simulink model "Copy_of_mavsim_chap10_model"  (R2020b)
settings: Solver=ode45  StartTime=0.0  StopTime=400  RelTol=1e-3  EnableMultiTasking=on
InitFcn:
  | param_chap10
undefined symbols (not defined in the file or in its folder): drawPathError, P, path_follow, path_manager_chap10
settings Model: Creator=beard  LastModifiedBy=彭美祥
settings DataIOCC: LimitDataPoints=on  SaveFormat=Array  SignalLoggingSaveFormat=ModelDataLogs  ReturnWorkspaceOutputs=off
settings OptimizationCC: ExpressionDepthLimit=2147483647  InitFltsAndDblsToZero=on  LifeSpan=inf
settings DebuggingCC: UnderspecifiedInitializationDetection=Classic  MergeDetectMultiDrivingBlocksExec=none  SolverPrmCheckMsg=warning  FcnCallInpInsideContextMsg=warning  StateNameClashWarn=warning  SFUnexpectedBacktrackingDiag=warning  SFNoUnconditionalDefaultTransitionDiag=warning  SFExecutionAtInitializationDiag=none  ArithmeticOperatorsInVariantConditions=warning
settings HardwareCC: ProdBitPerPointer=32  ProdBitPerSizeT=32  ProdBitPerPtrDiffT=32  ProdLargestAtomicFloat=None  ProdIntDivRoundTo=Undefined  ProdEndianess=Unspecified  ProdWordSize=32  ProdHWDeviceType=32-bit Generic
settings ModelReferenceCC: PropagateSignalLabelsOutOfModel=off
settings SFSimCC: SimUseLocalCustomCode=off  SimParseCustomCode=off  CustomCodeUndefinedFunction=UseInterfaceOnly
settings RTWCC: RTWUseLocalCustomCode=off
settings CodeAppCC: StateflowObjectComments=on
settings GRTTargetCC: TargetLangStandard=C89/C90 (ANSI)  CombineOutputUpdateFcns=off  GRTInterface=on
settings ConfigComp: CovMetricSettings=dw  CovSaveCumulativeToWorkspaceVar=on  CovSaveSingleToWorkspaceVar=on  CovExternalEMLEnable=off  CovSFcnEnable=off

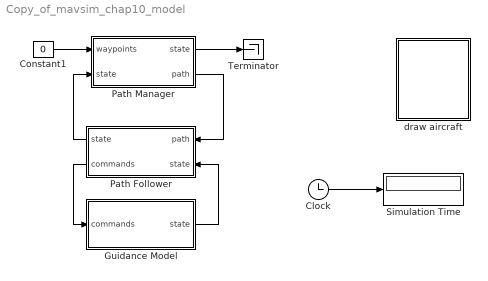
== system Copy_of_mavsim_chap10_model ==
  Clock : Clock
  Constant1 : Constant  Value=0
  Guidance Model : Subsystem
  Path Follower : Subsystem
  Path Manager : Subsystem
  Simulation Time : Display
  Terminator : Terminator
  draw aircraft : Subsystem
      mask Display: image(imread('tv.jpg'))
  wires:
  Clock/1 -> Simulation Time/1
  Path Manager/2(path) -> Path Follower/1(path)
  Path Follower/2(commands) -> Guidance Model/1(commands)
  Guidance Model/1(state) -> Path Follower/2(state)
  Constant1/1 -> Path Manager/1(waypoints)
  Path Follower/1("state ") -> Path Manager/2(state)
  Path Manager/1("state ") -> Terminator/1

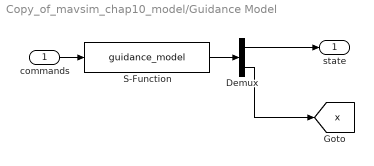
== system Copy_of_mavsim_chap10_model/Guidance Model ==
  commands : Inport
  Demux : Demux  Outputs=[16;12]
  S-Function : S-Function  FunctionName=guidance_model  Parameters=P  SFunctionDeploymentMode=off  EnableBusSupport=off
  state : Outport
  tag scope: x=global
  wires:
  commands/1 -> S-Function/1
  S-Function/1 -> Demux/1
  Demux/1 -> state/1
  Demux/2 -> [x]

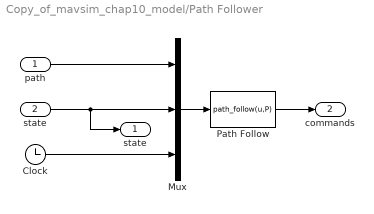
== system Copy_of_mavsim_chap10_model/Path Follower ==
  path : Inport
  state : Inport  Port=2
  Clock : Clock
  Mux : Mux  Inputs=3
  Path Follow : MATLABFcn  MATLABFcn=path_follow(u,P)  OutputDimensions=3  SampleTime=P.Ts
  "state " : Outport
  commands : Outport  Port=2
  wires:
  Path Follow/1 -> commands/1
  Mux/1 -> Path Follow/1
  path/1 -> Mux/1
  Clock/1 -> Mux/3
  state/1 -> Mux/2, "state "/1

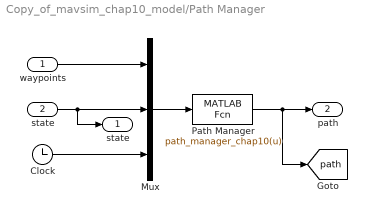
== system Copy_of_mavsim_chap10_model/Path Manager ==
  waypoints : Inport
  state : Inport  Port=2
  Clock : Clock
  Mux : Mux  Inputs=3
  Path Manager : MATLABFcn  MATLABFcn=path_manager_chap10(u)  OutputDimensions=13  SampleTime=P.Ts
  "state " : Outport
  path : Outport  Port=2
  tag scope: path=global
  wires:
  Path Manager/1 -> path/1, [path]
  Mux/1 -> Path Manager/1
  Clock/1 -> Mux/3
  state/1 -> Mux/2, "state "/1
  waypoints/1 -> Mux/1

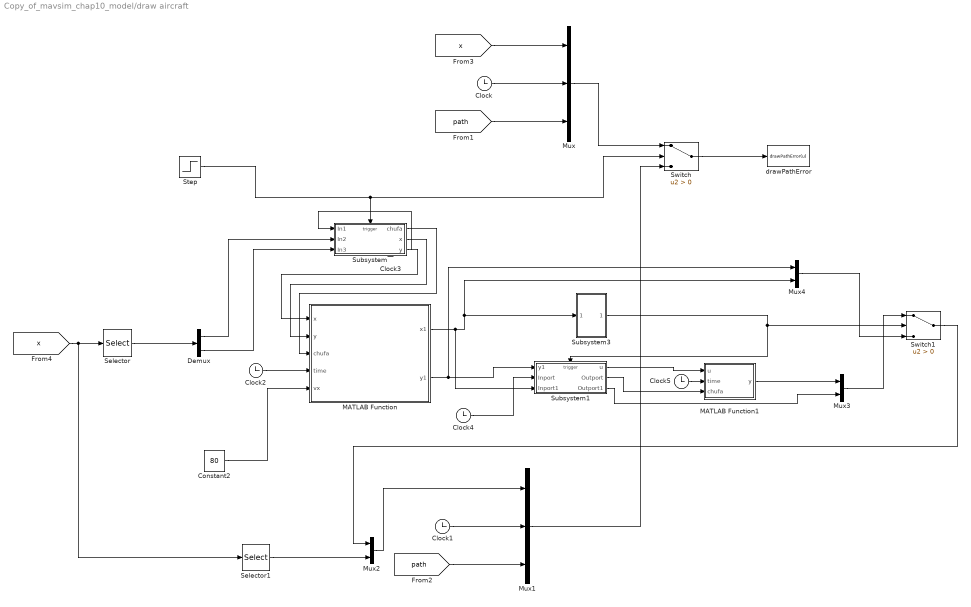
== system Copy_of_mavsim_chap10_model/draw aircraft ==
  Clock{,1..5} (6 alike) : Clock
  Constant2 : Constant  Value=80
  Demux : Demux  Outputs=2
  MATLAB Function : MATLAB Function  TreatAsAtomicUnit=on
  MATLAB Function1 : MATLAB Function  TreatAsAtomicUnit=on
  Mux : Mux  Inputs=3
  Mux1 : Mux  Inputs=3
  Mux2 : Mux  Inputs=2
  Mux3 : Mux  Inputs=2
  Mux4 : Mux  Inputs=2
  Selector : Selector  InputPortWidth=12  IndexOptions=Index vector (dialog)  Indices=[1 2]  OutputSizes=1
  Selector1 : Selector  InputPortWidth=12  IndexOptions=Index vector (dialog)  Indices=[3:12]  OutputSizes=1
  Step : Step  Time=176  Before=1  After=0  SampleTime=0
  Subsystem : Subsystem
  Subsystem1 : Subsystem
  Subsystem3 : Subsystem
  Switch : Switch  Criteria=u2 > Threshold
  Switch1 : Switch  Criteria=u2 > Threshold
  drawPathError : MATLABFcn  MATLABFcn=drawPathError(u)  OutputDimensions=0  SampleTime=0.1
  wires:
  Clock/1 -> Mux/2
  [x] -> Mux/1
  [path] -> Mux/3
  Step/1 -> Switch/2, Subsystem/Trigger
  Mux/1 -> Switch/1
  Switch/1 -> drawPathError/1
  Mux1/1 -> Switch/3
  Clock1/1 -> Mux1/2
  [path] -> Mux1/3
  [x] -> Selector1/1, Selector/1
  Selector/1 -> Demux/1
  Clock2/1 -> MATLAB Function/4(time)
  Clock3/1 -> Subsystem/1(In1)
  Subsystem/1(chufa) -> MATLAB Function/3(chufa)
  Constant2/1 -> MATLAB Function/5(vx)
  Demux/1 -> Subsystem/2(In2)
  Demux/2 -> Subsystem/3(In3)
  Subsystem/2(x) -> MATLAB Function/2(y)
  Subsystem/3(y) -> MATLAB Function/1(x)
  Mux2/1 -> Mux1/1
  MATLAB Function/1(x1) -> Subsystem1/3(Inport1), Subsystem3/1(In1), Mux4/2
  MATLAB Function/2(y1) -> Mux4/1, Subsystem1/1(y1)
  Clock4/1 -> Subsystem1/2(Inport)
  Subsystem1/1(u) -> MATLAB Function1/1(u)
  Clock5/1 -> MATLAB Function1/2(time)
  Subsystem1/2(Outport) -> MATLAB Function1/3(chufa)
  Selector1/1 -> Mux2/2
  MATLAB Function1/1(y) -> Mux3/1
  Subsystem1/3(Outport1) -> Mux3/2
  Switch1/1 -> Mux2/1
  Mux4/1 -> Switch1/3
  Mux3/1 -> Switch1/1
  Subsystem3/1(Out1) -> Subsystem1/Trigger, Switch1/2

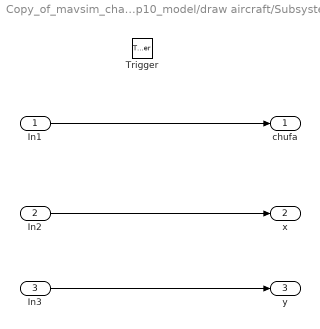
== system Copy_of_mavsim_chap10_model/draw aircraft/Subsystem ==
  In1 : Inport
  In2 : Inport  Port=2
  In3 : Inport  Port=3
  Trigger : TriggerPort  TriggerType=falling  VariantControl=Variant  PortDimensions=1
  chufa : Outport
  x : Outport  Port=2
  y : Outport  Port=3
  wires:
  In1/1 -> chufa/1
  In2/1 -> x/1
  In3/1 -> y/1

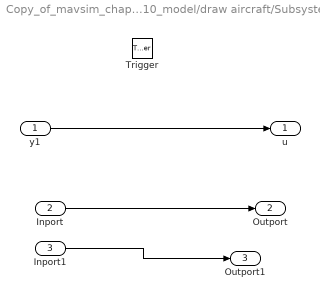
== system Copy_of_mavsim_chap10_model/draw aircraft/Subsystem1 ==
  y1 : Inport
  Inport : Inport  Port=2
  Inport1 : Inport  Port=3
  Trigger : TriggerPort  VariantControl=Variant  PortDimensions=1
  u : Outport
  Outport : Outport  Port=2
  Outport1 : Outport  Port=3
  wires:
  y1/1 -> u/1
  Inport/1 -> Outport/1
  Inport1/1 -> Outport1/1

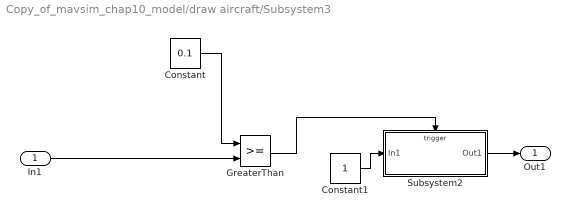
== system Copy_of_mavsim_chap10_model/draw aircraft/Subsystem3 ==
  In1 : Inport
  Constant : Constant  Value=0.1
  Constant1 : Constant
  GreaterThan : RelationalOperator  OutDataTypeStr=boolean  RndMeth=Simplest
  Subsystem2 : Subsystem
  Out1 : Outport
  wires:
  GreaterThan/1 -> Subsystem2/Trigger
  Constant1/1 -> Subsystem2/1(In1)
  Constant/1 -> GreaterThan/1
  Subsystem2/1(Out1) -> Out1/1
  In1/1 -> GreaterThan/2

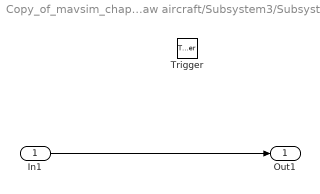
== system Copy_of_mavsim_chap10_model/draw aircraft/Subsystem3/Subsystem2 ==
  In1 : Inport
  Trigger : TriggerPort  VariantControl=Variant  PortDimensions=1
  Out1 : Outport
  wires:
  In1/1 -> Out1/1

== matlab function Copy_of_mavsim_chap10_model/draw aircraft/MATLAB Function1 ==
  data: u input; y output; time input; chufa input
function y = fcn(u,time,chufa)

y = u + 40*(time - chufa);

== matlab function Copy_of_mavsim_chap10_model/draw aircraft/MATLAB Function ==
  data: x input; x1 output; y input; chufa input; time input; vx input; y1 output
function [x1,y1] = tuning2landing(x,y,chufa,time,vx)
angle = atan(-x/y);
theta = pi/2 - angle;
AB = 800*(-x/y);
r = AB * tan(theta/2);
Ox1 = r;
Oy1 = Ox1* y/x;
w = vx / r;
t = time-chufa;
angle1 = angle-pi/2 - w*t;
x1 = Ox1 + r*cos(angle1);
y1 = Oy1 + r*sin(angle1);


end
